simulink model "HybridControllerD3D3"  (Simulink 8.2)
settings: Solver=FixedStepDiscrete  StartTime=0.0  StopTime=inf  RelTol=1e-3
PreLoadFcn:
  | initializeSimulation
  | initializeSCRAMNetGT
values from neighbouring files (symbols this model uses):
  node = scgtnodestruct(node)    [initializeSCRAMNetGT.m]
undefined symbols (not defined in the file or in its folder): nAcc, nAct, nAdcU, nDucU, nTbl
undefined symbols (not defined in the file): controlPeriod, HybridCtrlParameters
libraries: xpclib x13, cwcec_scgtLib x7, simulink x4
CloseFcn:
  | rtwprivate ssgencode ModelCloseRequest scrnet_receiver
settings Model: Creator=aschellenberg  LastModifiedBy=RTHS Analyst  ExtModeArmWhenConnect=off  BufferReuse=off
settings DataIOCC: LimitDataPoints=off  SignalLoggingSaveFormat=Dataset  SaveOutput=off  SignalLogging=off  SaveTime=off  SignalLoggingName=sigsOut
settings OptimizationCC: BlockReduction=off  OptimizeBlockIOStorage=off  BufferReuse=off  ExpressionFolding=off  FoldNonRolledExpr=off  LocalBlockOutputs=off  UseTempVars=on  InitFltsAndDblsToZero=on  EfficientFloat2IntCast=on  SimCompilerOptimization=On
settings DebuggingCC: SaveWithParameterizedLinksMsg=none  CheckSSInitialOutputMsg=off  SolverPrmCheckMsg=none  FcnCallInpInsideContextMsg=EnableAllAsError
settings HardwareCC: ProdIntDivRoundTo=Zero  ProdEndianess=LittleEndian  ProdHWDeviceType=Generic->32-bit x86 compatible  TargetHWDeviceType=32-bit Generic
settings SFSimCC: SimCustomHeaderCode="#include \"PredictorCorrector.h\""  SimUserSources=PredictorCorrector.c  SimUserIncludeDirs="\"C:\\Program Files\\OpenFresco\\SourceCode\\SRC\\experimentalControl\\Simulink\\HybridSimToolbox\""
settings RTWCC: SystemTargetFile=xpctarget.tlc  TemplateMakefile=xpc_default_tmf  Description=xPC Target  ProcessScript=xpctarget_make_rtw_hook  CustomHeaderCode="#include \"PredictorCorrector.h\""  CustomInclude="\"C:\\Program Files\\OpenFresco\\SourceCode\\SRC\\experimentalControl\\Simulink\\HybridSimToolbox\""  CustomSource=PredictorCorrector.c  IncludeERTFirstTime=on  RTWCompilerOptimization=On
settings xpcTargetCC: TargetFcnLib=ansi_tfl_tmw.mat  CodeReplacementLibrary=XPC_BLAS  ParMdlRefBuildCompliant=on  ConcurrentExecutionCompliant=on  CombineSignalStateStructs=off  MATLABClassNameForMDSCustomization=xpcAperiodicCustomization  GRTInterface=on  GenerateAllocFcn=off  xPCTaskExecutionProfile=off  xPCRL32EventNumber=5000  RL32IRQSourceModifier=Auto (PCI only)  xPCIRQSourceBoard=SCRAMNet_GT200  xPCLoadParamSetFile=off  xPCConcurrentTasks=off  xPCEnableSFAnimation=off

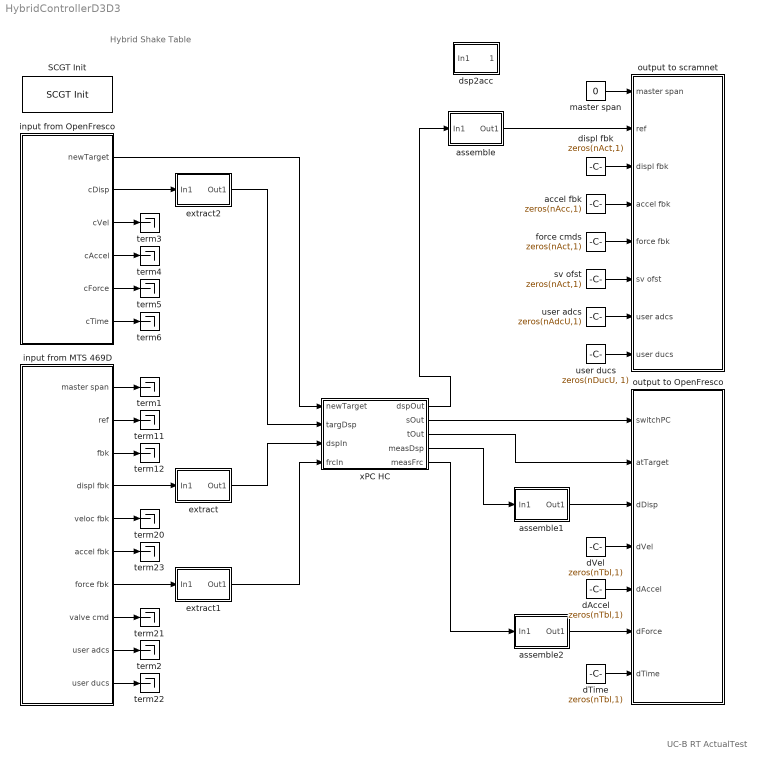
== system HybridControllerD3D3 ==
  note: Hybrid Shake Table
  note: UC-B RT ActualTest
  "SCGT Init " : cwcec_scgtLib/SCGT Init   node=node  pci=-1
  accel fbk : Constant  Value=zeros(nAcc,1)
  assemble : Subsystem  mask(to Actuators){id=[1], size=nTbl}
      mask prompts: id "Index Vector: id"; size "Vector Size: size"
      mask help: To select to which actuator(s) the signals are going to
      mask Display: disp('Assemble')
  assemble1 : Subsystem  mask(to Actuators){id=[1], size=nTbl}
      mask prompts: id "Index Vector: id"; size "Vector Size: size"
      mask help: To select to which actuator(s) the signals are going to
      mask Display: disp('Assemble')
  assemble2 : Subsystem  mask(to Actuators){id=[1], size=nTbl}
      mask prompts: id "Index Vector: id"; size "Vector Size: size"
      mask help: To select to which actuator(s) the signals are going to
      mask Display: disp('Assemble')
  dAccel : Constant  Value=zeros(nTbl,1)
  dTime : Constant  Value=zeros(nTbl,1)
  dVel : Constant  Value=zeros(nTbl,1)
  displ fbk : Constant  Value=zeros(nAct,1)
  dsp2acc : Subsystem
  extract : Subsystem  mask(from Actuators){id=[1], size=nTbl}
      mask prompts: id "Index Vector: id"; size "Vector Size: size"
      mask help: To select from which actuator(s) the signals are coming from
      mask Display: disp('Extract')
  extract1 : Subsystem  mask(from Actuators){id=[1], size=nTbl}
      mask prompts: id "Index Vector: id"; size "Vector Size: size"
      mask help: To select from which actuator(s) the signals are coming from
      mask Display: disp('Extract')
  extract2 : Subsystem  mask(from Actuators){id=[1], size=nTbl}
      mask prompts: id "Index Vector: id"; size "Vector Size: size"
      mask help: To select from which actuator(s) the signals are coming from
      mask Display: disp('Extract')
  force cmds : Constant  Value=zeros(nAct,1)
  input from MTS 469D : Subsystem
  input from OpenFresco : Subsystem
  master span : Constant  Value=0
  output to OpenFresco : Subsystem
  output to scramnet : Subsystem
  sv ofst : Constant  Value=zeros(nAct,1)
  term{1..6,11..12,20..23} (12 alike) : Terminator
  user adcs : Constant  Value=zeros(nAdcU,1)
  user ducs : Constant  Value=zeros(nDucU, 1)  OutDataTypeStr=uint32
  xPC HC : Subsystem  mask(Hybrid Controller: D3/D3){nAct=1, dtInt=HybridCtrlParameters.dtInt, dtSim=HybridCtrlParameters.dtSim, dtCon=HybridCtrlParameters.dtCon, N=HybridCtrlParameters.N, iDelay=HybridCtrlParameters.iDelay}
      mask prompts: nAct "Number of Actuators: nAct"; dtInt "Integration time step: dtInt"; dtSim "Simulation time step: dtSim"; dtCon "Controller time step: dtCon"; N "Maximum number of substeps: N"; iDelay "Number of delay steps: iDelay"
      mask help: Hybrid Controller using C0-continuous cubic Lagrange interpolation for prediction and correction
      mask Display: disp('xPC Target\nHybrid Controller\n(D3/D3)')
  wires:
  master span/1 -> output to scramnet/1(master span)
  force cmds/1 -> output to scramnet/5(force fbk)
  displ fbk/1 -> output to scramnet/3(displ fbk)
  user ducs/1 -> output to scramnet/8(user ducs)
  dVel/1 -> output to OpenFresco/4(dVel)
  dAccel/1 -> output to OpenFresco/5(dAccel)
  dTime/1 -> output to OpenFresco/7(dTime)
  input from OpenFresco/3(cVel) -> term3/1
  input from OpenFresco/5(cForce) -> term5/1
  input from OpenFresco/6(cTime) -> term6/1
  input from OpenFresco/1(newTarget) -> xPC HC/1(newTarget)
  extract2/1(Out1) -> xPC HC/2(targDsp)
  extract/1(Out1) -> xPC HC/3(dspIn)
  extract1/1(Out1) -> xPC HC/4(frcIn)
  xPC HC/1(dspOut) -> assemble/1(In1)
  xPC HC/5(measFrc) -> assemble2/1(In1)
  xPC HC/4(measDsp) -> assemble1/1(In1)
  xPC HC/3(tOut) -> output to OpenFresco/2(atTarget)
  xPC HC/2(sOut) -> output to OpenFresco/1(switchPC)
  assemble1/1(Out1) -> output to OpenFresco/3(dDisp)
  assemble2/1(Out1) -> output to OpenFresco/6(dForce)
  input from MTS 469D/1(master span) -> term1/1
  input from MTS 469D/2(ref) -> term11/1
  input from MTS 469D/3(fbk) -> term12/1
  input from MTS 469D/4(displ fbk) -> extract/1(In1)
  input from MTS 469D/5(veloc fbk) -> term20/1
  input from MTS 469D/6(accel fbk) -> term23/1
  input from MTS 469D/7(force fbk) -> extract1/1(In1)
  input from MTS 469D/8(valve cmd) -> term21/1
  input from MTS 469D/10(user ducs) -> term22/1
  input from MTS 469D/9(user adcs) -> term2/1
  accel fbk/1 -> output to scramnet/4(accel fbk)
  user adcs/1 -> output to scramnet/7(user adcs)
  input from OpenFresco/2(cDisp) -> extract2/1(In1)
  input from OpenFresco/4(cAccel) -> term4/1
  sv ofst/1 -> output to scramnet/6(sv ofst)
  assemble/1(Out1) -> output to scramnet/2(ref)

== system HybridControllerD3D3/assemble ==
  In1 : Inport
  Assignment : Assignment  OutputInitialize=Specify size for each dimension in table  IndexOptions=Index vector (port)  Indices=1  OutputSizes=size
  Constant : Constant  Value=id
  Out1 : Outport
  wires:
  Constant/1 -> Assignment/2
  Assignment/1 -> Out1/1
  In1/1 -> Assignment/1

== system HybridControllerD3D3/assemble1 ==
  In1 : Inport
  Assignment : Assignment  OutputInitialize=Specify size for each dimension in table  IndexOptions=Index vector (port)  Indices=1  OutputSizes=size
  Constant : Constant  Value=id
  Out1 : Outport
  wires:
  Constant/1 -> Assignment/2
  Assignment/1 -> Out1/1
  In1/1 -> Assignment/1

== system HybridControllerD3D3/assemble2 ==
  In1 : Inport
  Assignment : Assignment  OutputInitialize=Specify size for each dimension in table  IndexOptions=Index vector (port)  Indices=1  OutputSizes=size
  Constant : Constant  Value=id
  Out1 : Outport
  wires:
  Constant/1 -> Assignment/2
  Assignment/1 -> Out1/1
  In1/1 -> Assignment/1

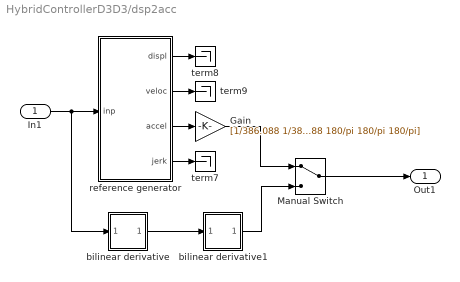
== system HybridControllerD3D3/dsp2acc ==
  In1 : Inport
  Gain : Gain  Gain=[1/386.088 1/386.088 1/386.088 180/pi 180/pi 180/pi]
  Manual Switch : ManualSwitch
  bilinear derivative : Subsystem  mask(Discrete Bilinear Differentiator){decay=1, initialCondition=0, samplePeriod=controlPeriod}
      mask prompts: decay "Decay time constant (0: backward Euler, 1: binlinear)"; initialCondition "Initial condition"; samplePeriod "Sample period"
      mask Display:
      | text(0.1,.75,'2');
      | text(0.1,.65,'_');
      | text(0.1,.25,'T');
      | text(.3,.80,'{1-z}^{-1}', 'hor','left','texmode','on');
      | text(.3,.65,'___');
      | text(.3,.30,'{1+z}^{-1}', 'hor','left','texmode','on');
  bilinear derivative1 : Subsystem  mask(Discrete Bilinear Differentiator){decay=1, initialCondition=0, samplePeriod=controlPeriod}
      mask prompts: decay "Decay time constant (0: backward Euler, 1: binlinear)"; initialCondition "Initial condition"; samplePeriod "Sample period"
      mask Display:
      | text(0.1,.75,'2');
      | text(0.1,.65,'_');
      | text(0.1,.25,'T');
      | text(.3,.80,'{1-z}^{-1}', 'hor','left','texmode','on');
      | text(.3,.65,'___');
      | text(.3,.30,'{1+z}^{-1}', 'hor','left','texmode','on');
  reference generator : Subsystem  mask(Reference Generator){mode=1, freqHP=0.0625, freqLP=128, displCanon=1, velocCanon=1, accelCanon=1, jerkCanon=1, samplePeriod=controlPeriod}
      mask prompts: mode "Mode (1: displ, 2: veloc, 3: accel)"; freqHP "Cut-in frequency (Hz)"; freqLP "Cutoff frequency (Hz)"; displCanon "Canonical displacement units"; velocCanon "Canonical velocity units"; accelCanon "Canonical acceleration units"; jerkCanon "Canonical jerk units"; samplePeriod "Sample period (sec)"
      mask init:
      | omegaHP	= 2 * pi * freqHP;
      | omegaLP	= 2 * pi * freqLP;
      | if mode == 1
      | 	damp = 0.707106781186547;
      | 	b  = omegaLP * omegaLP;
      | 	a0 = 0;
      | 	a1 = omegaLP * omegaLP;
      | 	a2 = 2 * damp * omegaLP;
      | 	canon = displCanon;
      | elseif mode == 2
      | 	damp = 0.707106781186547;
      | 	b  = omegaLP;
      | 	a0 = omegaHP * omegaHP * omegaLP;
      | 	a1 = (2 * damp * omegaLP + omegaHP) * omegaHP;
      | 	a2 = 2 * damp * omegaHP + omegaLP;
      | 	canon = velocCanon;
      | elseif mode == 3
      | 	damp = 0.5;
      | 	b  = 1;
      | 	a0 = omegaHP * omegaHP * omegaHP;
      | 	a1 = (2 * damp + 1) * omegaHP * omegaHP;
      | 	a2 = (2 * damp + 1) * omegaHP;
      | 	canon = accelCanon;
      | end
  term7 : Terminator
  term8 : Terminator
  term9 : Terminator
  Out1 : Outport
  wires:
  In1/1 -> reference generator/1(inp), bilinear derivative/1(inp)
  reference generator/2(veloc) -> term9/1
  reference generator/4(jerk) -> term7/1
  reference generator/1(displ) -> term8/1
  reference generator/3(accel) -> Gain/1
  bilinear derivative/1(out) -> bilinear derivative1/1(inp)
  Gain/1 -> Manual Switch/1
  bilinear derivative1/1(out) -> Manual Switch/2
  Manual Switch/1 -> Out1/1

== system HybridControllerD3D3/extract ==
  In1 : Inport
  Selector : Selector  InputPortWidth=size  IndexOptions=Index vector (dialog)  Indices=id  OutputSizes=1
  Out1 : Outport
  wires:
  Selector/1 -> Out1/1
  In1/1 -> Selector/1

== system HybridControllerD3D3/extract1 ==
  In1 : Inport
  Selector : Selector  InputPortWidth=size  IndexOptions=Index vector (dialog)  Indices=id  OutputSizes=1
  Out1 : Outport
  wires:
  Selector/1 -> Out1/1
  In1/1 -> Selector/1

== system HybridControllerD3D3/extract2 ==
  In1 : Inport
  Selector : Selector  InputPortWidth=size  IndexOptions=Index vector (dialog)  Indices=id  OutputSizes=1
  Out1 : Outport
  wires:
  Selector/1 -> Out1/1
  In1/1 -> Selector/1

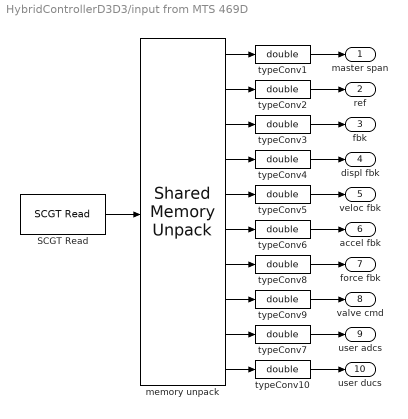
== system HybridControllerD3D3/input from MTS 469D ==
  "SCGT Read " : cwcec_scgtLib/SCGT Read   partition=node.Partitions(9:18)  ts=controlPeriod  pci=-1
  memory unpack : xpclib/Shared Memory/Shared Memory Unpack   partition=node.Partitions(9:18)
  typeConv{1..10} (10 alike) : DataTypeConversion  OutDataTypeStr=double  SaturateOnIntegerOverflow=on  RndMeth=Zero
  master span : Outport
  ref : Outport  Port=2
  fbk : Outport  Port=3
  displ fbk : Outport  Port=4
  veloc fbk : Outport  Port=5
  accel fbk : Outport  Port=6
  force fbk : Outport  Port=7
  valve cmd : Outport  Port=8
  user adcs : Outport  Port=9
  user ducs : Outport  Port=10
  wires:
  memory unpack/10 -> typeConv10/1
  memory unpack/9 -> typeConv7/1
  memory unpack/8 -> typeConv9/1
  memory unpack/7 -> typeConv8/1
  memory unpack/6 -> typeConv6/1
  memory unpack/5 -> typeConv5/1
  memory unpack/4 -> typeConv4/1
  memory unpack/3 -> typeConv3/1
  memory unpack/2 -> typeConv2/1
  memory unpack/1 -> typeConv1/1
  typeConv2/1 -> ref/1
  typeConv1/1 -> master span/1
  "SCGT Read "/1 -> memory unpack/1
  typeConv3/1 -> fbk/1
  typeConv4/1 -> displ fbk/1
  typeConv5/1 -> veloc fbk/1
  typeConv6/1 -> accel fbk/1
  typeConv8/1 -> force fbk/1
  typeConv9/1 -> valve cmd/1
  typeConv7/1 -> user adcs/1
  typeConv10/1 -> user ducs/1

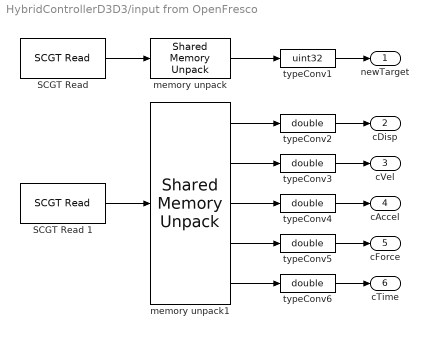
== system HybridControllerD3D3/input from OpenFresco ==
  "SCGT Read " : cwcec_scgtLib/SCGT Read   partition=node.Partitions(19)  ts=controlPeriod  pci=-1
  SCGT Read 1 : cwcec_scgtLib/SCGT Read   partition=node.Partitions(22:26)  ts=controlPeriod  pci=-1
  memory unpack : xpclib/Shared Memory/Shared Memory Unpack   partition=node.Partitions(19)
  memory unpack1 : xpclib/Shared Memory/Shared Memory Unpack   partition=node.Partitions(22:26)
  typeConv1 : DataTypeConversion  OutDataTypeStr=uint32  SaturateOnIntegerOverflow=on  RndMeth=Zero
  typeConv{2..6} (5 alike) : DataTypeConversion  OutDataTypeStr=double  SaturateOnIntegerOverflow=on  RndMeth=Zero
  newTarget : Outport
  cDisp : Outport  Port=2
  cVel : Outport  Port=3
  cAccel : Outport  Port=4
  cForce : Outport  Port=5
  cTime : Outport  Port=6
  wires:
  typeConv1/1 -> newTarget/1
  memory unpack/1 -> typeConv1/1
  typeConv2/1 -> cDisp/1
  typeConv3/1 -> cVel/1
  memory unpack1/2 -> typeConv3/1
  typeConv4/1 -> cAccel/1
  memory unpack1/3 -> typeConv4/1
  typeConv5/1 -> cForce/1
  typeConv6/1 -> cTime/1
  memory unpack1/5 -> typeConv6/1
  memory unpack1/4 -> typeConv5/1
  "SCGT Read "/1 -> memory unpack/1
  SCGT Read 1/1 -> memory unpack1/1
  memory unpack1/1 -> typeConv2/1

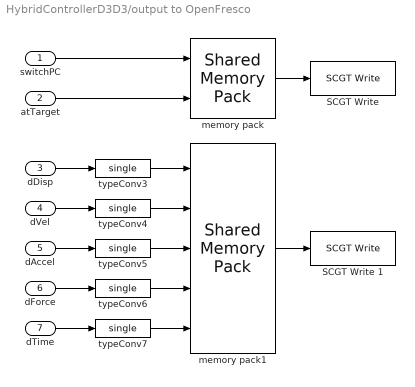
== system HybridControllerD3D3/output to OpenFresco ==
  switchPC : Inport
  atTarget : Inport  Port=2
  dDisp : Inport  Port=3
  dVel : Inport  Port=4
  dAccel : Inport  Port=5
  dForce : Inport  Port=6
  dTime : Inport  Port=7
  "SCGT Write " : cwcec_scgtLib/SCGT Write   partition=node.Partitions(20:21)  ts=controlPeriod  pci=-1
  SCGT Write 1 : cwcec_scgtLib/SCGT Write   partition=node.Partitions(27:31)  ts=controlPeriod  pci=-1
  memory pack : xpclib/Shared Memory/Shared Memory Pack   partition=node.Partitions(20:21)
  memory pack1 : xpclib/Shared Memory/Shared Memory Pack   partition=node.Partitions(27:31)
  typeConv{3..7} (5 alike) : DataTypeConversion  OutDataTypeStr=single  SaturateOnIntegerOverflow=on  RndMeth=Zero
  wires:
  dAccel/1 -> typeConv5/1
  switchPC/1 -> memory pack/1
  dVel/1 -> typeConv4/1
  dDisp/1 -> typeConv3/1
  typeConv4/1 -> memory pack1/2
  typeConv5/1 -> memory pack1/3
  dForce/1 -> typeConv6/1
  typeConv6/1 -> memory pack1/4
  dTime/1 -> typeConv7/1
  typeConv7/1 -> memory pack1/5
  atTarget/1 -> memory pack/2
  memory pack/1 -> "SCGT Write "/1
  memory pack1/1 -> SCGT Write 1/1
  typeConv3/1 -> memory pack1/1

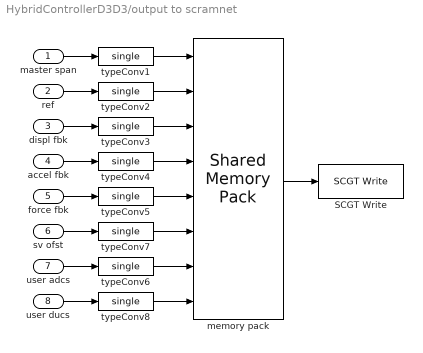
== system HybridControllerD3D3/output to scramnet ==
  master span : Inport
  ref : Inport  Port=2
  displ fbk : Inport  Port=3
  accel fbk : Inport  Port=4
  force fbk : Inport  Port=5
  sv ofst : Inport  Port=6
  user adcs : Inport  Port=7
  user ducs : Inport  Port=8
  "SCGT Write " : cwcec_scgtLib/SCGT Write   partition=node.Partitions(1:8)  ts=controlPeriod  pci=-1
  memory pack : xpclib/Shared Memory/Shared Memory Pack   partition=node.Partitions(1:8)
  typeConv{1..8} (8 alike) : DataTypeConversion  OutDataTypeStr=single  SaturateOnIntegerOverflow=on  RndMeth=Zero
  wires:
  typeConv8/1 -> memory pack/8
  user ducs/1 -> typeConv8/1
  user adcs/1 -> typeConv6/1
  sv ofst/1 -> typeConv7/1
  master span/1 -> typeConv1/1
  ref/1 -> typeConv2/1
  displ fbk/1 -> typeConv3/1
  accel fbk/1 -> typeConv4/1
  memory pack/1 -> "SCGT Write "/1
  typeConv1/1 -> memory pack/1
  typeConv2/1 -> memory pack/2
  typeConv3/1 -> memory pack/3
  typeConv4/1 -> memory pack/4
  force fbk/1 -> typeConv5/1
  typeConv5/1 -> memory pack/5
  typeConv7/1 -> memory pack/6
  typeConv6/1 -> memory pack/7

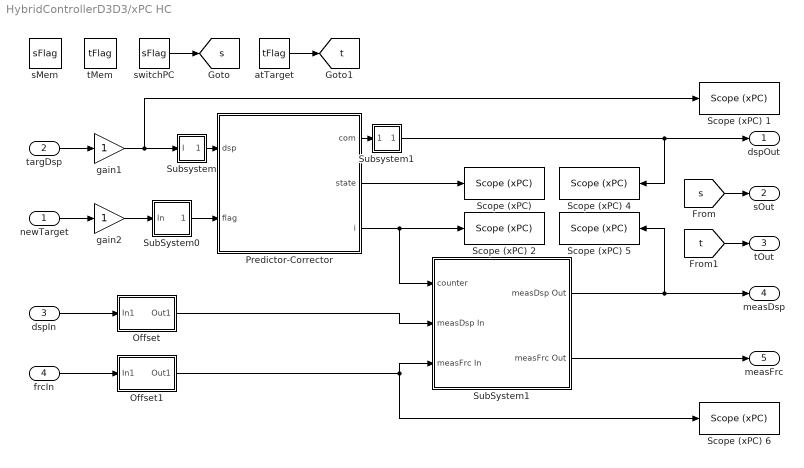
== system HybridControllerD3D3/xPC HC ==
  newTarget : Inport
  targDsp : Inport  Port=2
  dspIn : Inport  Port=3
  frcIn : Inport  Port=4
  Offset : Subsystem  mask(Signal Offset){nS=nAct, nOffset=1/dtCon, dt=dtCon}
      mask prompts: nS "Number of Signals: nS"; nOffset "Number of samples to initialize offset: nOffset"; dt "Sample time: dt"
      mask help: Offset signal by average of signal over initial number of samples
      mask Display: fprintf('Signal\nOffset')
  Offset1 : Subsystem  mask(Signal Offset){nS=nAct, nOffset=1/dtCon, dt=dtCon}
      mask prompts: nS "Number of Signals: nS"; nOffset "Number of samples to initialize offset: nOffset"; dt "Sample time: dt"
      mask help: Offset signal by average of signal over initial number of samples
      mask Display: fprintf('Signal\nOffset')
  Predictor-Corrector : Stateflow chart  TreatAsAtomicUnit=on
  "Scope (xPC) " : xpclib/Misc./Scope (xPC)   scopeno=4  scopetype=File  autostart=on  viewmode=Graphical redraw  formatstr='%15.6f'  grid=on  ylimits=[0,3]  nosamples=4096  noprepostsamples=0  interleave=1  triggermode=FreeRun  triggersignal=1  trigsignalfromport=off  triggerlevel=0.0  triggerslope=Either  triggerscope=1  triggersample=0  filename=D:\state.dat  mode=Lazy  writesize=512  autorestart=on  dynamicfilemode=off  maxwritefilesize=512*1024^2
  Scope (xPC) 1 : xpclib/Misc./Scope (xPC)   scopeno=1  scopetype=File  autostart=on  viewmode=Numerical  formatstr='%15.6f'  grid=on  ylimits=[-4,4]  nosamples=4096  noprepostsamples=0  interleave=1  triggermode=FreeRun  triggersignal=1  trigsignalfromport=off  triggerlevel=0.0  triggerslope=Either  triggerscope=1  triggersample=0  filename=D:\targDsp.dat  mode=Lazy  writesize=512  autorestart=on  dynamicfilemode=off  maxwritefilesize=512*1024^2
  Scope (xPC) 2 : xpclib/Misc./Scope (xPC)   scopeno=5  scopetype=File  autostart=on  viewmode=Numerical  formatstr='%15.6f'  grid=on  ylimits=[0,3]  nosamples=4096  noprepostsamples=0  interleave=1  triggermode=FreeRun  triggersignal=1  trigsignalfromport=off  triggerlevel=0.0  triggerslope=Either  triggerscope=1  triggersample=0  filename=D:\count.dat  mode=Lazy  writesize=512  autorestart=on  dynamicfilemode=off  maxwritefilesize=512*1024^2
  Scope (xPC) 4 : xpclib/Misc./Scope (xPC)   scopeno=2  scopetype=File  autostart=on  viewmode=Numerical  formatstr='%15.6f'  grid=on  ylimits=[-4,4]  nosamples=4096  noprepostsamples=0  interleave=1  triggermode=FreeRun  triggersignal=1  trigsignalfromport=off  triggerlevel=0.0  triggerslope=Either  triggerscope=1  triggersample=0  filename=D:\commDsp.dat  mode=Lazy  writesize=512  autorestart=on  dynamicfilemode=off  maxwritefilesize=512*1024^2
  Scope (xPC) 5 : xpclib/Misc./Scope (xPC)   scopeno=3  scopetype=File  autostart=on  viewmode=Numerical  formatstr='%15.6f'  grid=on  ylimits=[-4,4]  nosamples=4096  noprepostsamples=0  interleave=1  triggermode=FreeRun  triggersignal=1  trigsignalfromport=off  triggerlevel=0.0  triggerslope=Either  triggerscope=1  triggersample=0  filename=D:\measDsp.dat  mode=Lazy  writesize=512  autorestart=on  dynamicfilemode=off  maxwritefilesize=512*1024^2
  Scope (xPC) 6 : xpclib/Misc./Scope (xPC)   scopeno=6  scopetype=File  autostart=on  viewmode=Numerical  formatstr='%15.6f'  grid=on  ylimits=[0,3]  nosamples=4096  noprepostsamples=0  interleave=1  triggermode=FreeRun  triggersignal=1  trigsignalfromport=off  triggerlevel=0.0  triggerslope=Either  triggerscope=1  triggersample=0  filename=D:\measFrc.dat  mode=Lazy  writesize=512  autorestart=on  dynamicfilemode=off  maxwritefilesize=512*1024^2
  SubSystem0 : Subsystem
  SubSystem1 : Subsystem
  Subsystem : Subsystem
      mask Display: disp('I/O')
  Subsystem1 : Subsystem
      mask Display: disp('I/O')
  atTarget : DataStoreRead  DataStoreName=tFlag  SampleTime=dtCon
  gain1 : Gain  OutDataTypeStr=Inherit: Same as input
  gain2 : Gain  OutDataTypeStr=Inherit: Same as input  ParamDataTypeStr=Inherit: Same as input
  sMem : DataStoreMemory  DataStoreName=sFlag  OutDataTypeStr=uint32
  switchPC : DataStoreRead  DataStoreName=sFlag  SampleTime=dtCon
  tMem : DataStoreMemory  DataStoreName=tFlag  OutDataTypeStr=uint32
  dspOut : Outport
  sOut : Outport  Port=2
  tOut : Outport  Port=3
  measDsp : Outport  Port=4
  measFrc : Outport  Port=5
  tag scope: s=global, t=global
  wires:
  frcIn/1 -> Offset1/1(In1)
  dspIn/1 -> Offset/1(In1)
  SubSystem1/2(measFrc Out) -> measFrc/1
  SubSystem1/1(measDsp Out) -> Scope (xPC) 5/1, measDsp/1
  Predictor-Corrector/3(i) -> SubSystem1/1(counter), Scope (xPC) 2/1
  Predictor-Corrector/2(state) -> "Scope (xPC) "/1
  Predictor-Corrector/1(com) -> Subsystem1/1(In)
  Offset/1(Out1) -> SubSystem1/2(measDsp In)
  SubSystem0/1(Out) -> Predictor-Corrector/2(flag)
  newTarget/1 -> gain2/1
  switchPC/1 -> [s]
  atTarget/1 -> [t]
  targDsp/1 -> gain1/1
  Offset1/1(Out1) -> Scope (xPC) 6/1, SubSystem1/3(measFrc In)
  [s] -> sOut/1
  [t] -> tOut/1
  gain1/1 -> Scope (xPC) 1/1, Subsystem/1(I)
  gain2/1 -> SubSystem0/1(In)
  Subsystem1/1(Out) -> Scope (xPC) 4/1, dspOut/1
  Subsystem/1(O) -> Predictor-Corrector/1(dsp)

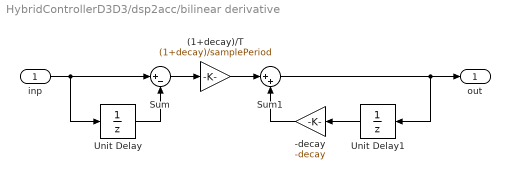
== system HybridControllerD3D3/dsp2acc/bilinear derivative ==
  inp : Inport
  (1+decay)/T : Gain  Gain=(1+decay)/samplePeriod
  -decay : Gain  Gain=-decay
  Sum : Sum  Inputs=|+-  SaturateOnIntegerOverflow=on  InputSameDT=on  OutDataTypeStr=Inherit: Same as first input
  Sum1 : Sum  Inputs=|++  SaturateOnIntegerOverflow=on  InputSameDT=on  OutDataTypeStr=Inherit: Same as first input
  Unit Delay : UnitDelay  InitialCondition=initialCondition  SampleTime=-1
  Unit Delay1 : UnitDelay  SampleTime=-1
  out : Outport
  wires:
  Sum/1 -> (1+decay)/T/1
  Unit Delay1/1 -> -decay/1
  inp/1 -> Sum/1, Unit Delay/1
  Unit Delay/1 -> Sum/2
  -decay/1 -> Sum1/2
  Sum1/1 -> out/1, Unit Delay1/1
  (1+decay)/T/1 -> Sum1/1

== system HybridControllerD3D3/dsp2acc/bilinear derivative1 ==
  inp : Inport
  (1+decay)/T : Gain  Gain=(1+decay)/samplePeriod
  -decay : Gain  Gain=-decay
  Sum : Sum  Inputs=|+-  SaturateOnIntegerOverflow=on  InputSameDT=on  OutDataTypeStr=Inherit: Same as first input
  Sum1 : Sum  Inputs=|++  SaturateOnIntegerOverflow=on  InputSameDT=on  OutDataTypeStr=Inherit: Same as first input
  Unit Delay : UnitDelay  InitialCondition=initialCondition  SampleTime=-1
  Unit Delay1 : UnitDelay  SampleTime=-1
  out : Outport
  wires:
  Sum/1 -> (1+decay)/T/1
  Unit Delay1/1 -> -decay/1
  inp/1 -> Sum/1, Unit Delay/1
  Unit Delay/1 -> Sum/2
  -decay/1 -> Sum1/2
  Sum1/1 -> out/1, Unit Delay1/1
  (1+decay)/T/1 -> Sum1/1

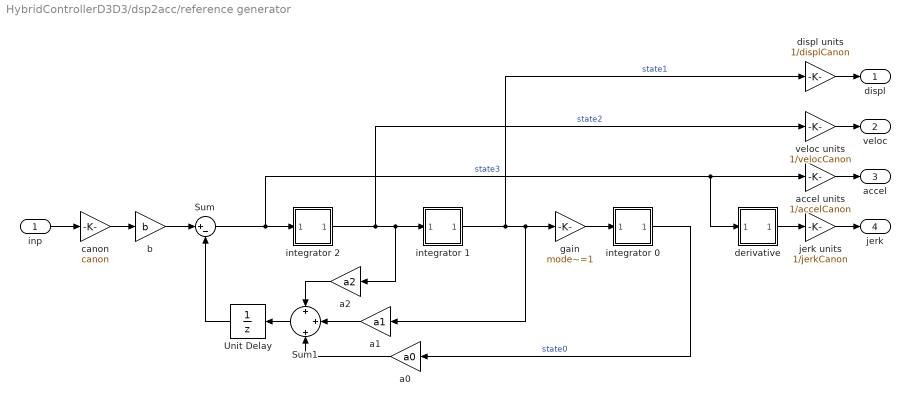
== system HybridControllerD3D3/dsp2acc/reference generator ==
  inp : Inport
  Sum : Sum  Inputs=|+-
  Sum1 : Sum  Inputs=+|+|+
  Unit Delay : UnitDelay  SampleTime=-1
  a0 : Gain  Gain=a0
  a1 : Gain  Gain=a1
  a2 : Gain  Gain=a2
  accel units : Gain  Gain=1/accelCanon
  b : Gain  Gain=b
  canon : Gain  Gain=canon
  derivative : Subsystem  mask(Discrete Euler Derivative){initialCondition=0, samplePeriod=samplePeriod}
      mask prompts: initialCondition "Initial condition"; samplePeriod "Sample period (sec)"
      mask Display: dpoly([1 -1], '[T]', 'z-')
  displ units : Gain  Gain=1/displCanon
  gain : Gain  Gain=mode~=1
  integrator 0 : Subsystem  mask(Discrete Bilinear Integrator){initialCondition=0, samplePeriod=samplePeriod}
      mask prompts: initialCondition "Initial condition"; samplePeriod "Sample period (sec)"
      mask Display:
      | text(0.1,.75,'T');
      | text(0.1,.65,'_');
      | text(0.1,.25,'2');
      | text(.3,.80,'{1+z}^{-1}', 'hor','left','texmode','on');
      | text(.3,.65,'___');
      | text(.3,.30,'{1-z}^{-1}', 'hor','left','texmode','on');
  integrator 1 : Subsystem  mask(Discrete Bilinear Integrator){initialCondition=0, samplePeriod=samplePeriod}
      mask prompts: initialCondition "Initial condition"; samplePeriod "Sample period (sec)"
      mask Display:
      | text(0.1,.75,'T');
      | text(0.1,.65,'_');
      | text(0.1,.25,'2');
      | text(.3,.80,'{1+z}^{-1}', 'hor','left','texmode','on');
      | text(.3,.65,'___');
      | text(.3,.30,'{1-z}^{-1}', 'hor','left','texmode','on');
  integrator 2 : Subsystem  mask(Discrete Bilinear Integrator){initialCondition=0, samplePeriod=samplePeriod}
      mask prompts: initialCondition "Initial condition"; samplePeriod "Sample period (sec)"
      mask Display:
      | text(0.1,.75,'T');
      | text(0.1,.65,'_');
      | text(0.1,.25,'2');
      | text(.3,.80,'{1+z}^{-1}', 'hor','left','texmode','on');
      | text(.3,.65,'___');
      | text(.3,.30,'{1-z}^{-1}', 'hor','left','texmode','on');
  jerk units : Gain  Gain=1/jerkCanon
  veloc units : Gain  Gain=1/velocCanon
  displ : Outport
  veloc : Outport  Port=2
  accel : Outport  Port=3
  jerk : Outport  Port=4
  wires:
  gain/1 -> integrator 0/1(inp)
  derivative/1(out) -> jerk units/1
  Unit Delay/1 -> Sum/2
  jerk units/1 -> jerk/1
  canon/1 -> b/1
  displ units/1 -> displ/1
  veloc units/1 -> veloc/1
  accel units/1 -> accel/1
  inp/1 -> canon/1
  integrator 0/1(out) -> a0/1  "state0"
  a0/1 -> Sum1/3
  a1/1 -> Sum1/2
  a2/1 -> Sum1/1
  Sum1/1 -> Unit Delay/1
  b/1 -> Sum/1
  Sum/1 -> integrator 2/1(inp), derivative/1(inp), accel units/1  "state3"
  integrator 1/1(out) -> displ units/1, gain/1, a1/1  "state1"
  integrator 2/1(out) -> veloc units/1, integrator 1/1(inp), a2/1  "state2"

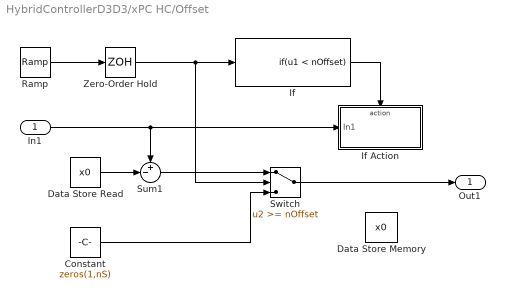
== system HybridControllerD3D3/xPC HC/Offset ==
  In1 : Inport
  Constant : Constant  Value=zeros(1,nS)
  Data Store Memory : DataStoreMemory  DataStoreName=x0  InitialValue=zeros(1,nS)  OutDataTypeStr=double
  Data Store Read : DataStoreRead  DataStoreName=x0  SampleTime=dt
  If : If  IfExpression=u1 < nOffset  ShowElse=off
  If Action : Subsystem  TreatAsAtomicUnit=on
  Ramp : simulink/Sources/Ramp  slope=1/dt  start=0  X0=0
  Sum1 : Sum  Inputs=+-|  SaturateOnIntegerOverflow=on  InputSameDT=on  OutDataTypeStr=Inherit: Same as first input
  Switch : Switch  Threshold=nOffset  SaturateOnIntegerOverflow=on  InputSameDT=on
  Zero-Order Hold : ZeroOrderHold  SampleTime=dt
  Out1 : Outport
  wires:
  Switch/1 -> Out1/1
  Sum1/1 -> Switch/1
  Data Store Read/1 -> Sum1/2
  In1/1 -> If Action/1(In1), Sum1/1
  Constant/1 -> Switch/3
  Zero-Order Hold/1 -> Switch/2, If/1
  If/1 -> If Action/Action
  Ramp/1 -> Zero-Order Hold/1

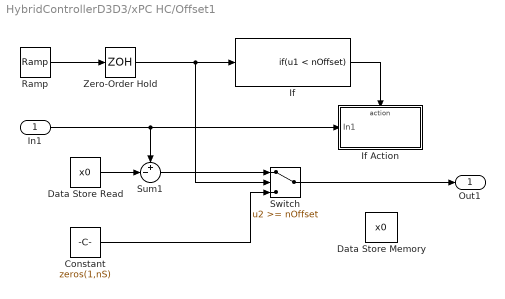
== system HybridControllerD3D3/xPC HC/Offset1 ==
  In1 : Inport
  Constant : Constant  Value=zeros(1,nS)
  Data Store Memory : DataStoreMemory  DataStoreName=x0  InitialValue=zeros(1,nS)  OutDataTypeStr=double
  Data Store Read : DataStoreRead  DataStoreName=x0  SampleTime=dt
  If : If  IfExpression=u1 < nOffset  ShowElse=off
  If Action : Subsystem  TreatAsAtomicUnit=on
  Ramp : simulink/Sources/Ramp  slope=1/dt  start=0  X0=0
  Sum1 : Sum  Inputs=+-|  SaturateOnIntegerOverflow=on  InputSameDT=on  OutDataTypeStr=Inherit: Same as first input
  Switch : Switch  Threshold=nOffset  SaturateOnIntegerOverflow=on  InputSameDT=on
  Zero-Order Hold : ZeroOrderHold  SampleTime=dt
  Out1 : Outport
  wires:
  Switch/1 -> Out1/1
  Sum1/1 -> Switch/1
  Data Store Read/1 -> Sum1/2
  In1/1 -> If Action/1(In1), Sum1/1
  Constant/1 -> Switch/3
  Zero-Order Hold/1 -> Switch/2, If/1
  If/1 -> If Action/Action
  Ramp/1 -> Zero-Order Hold/1

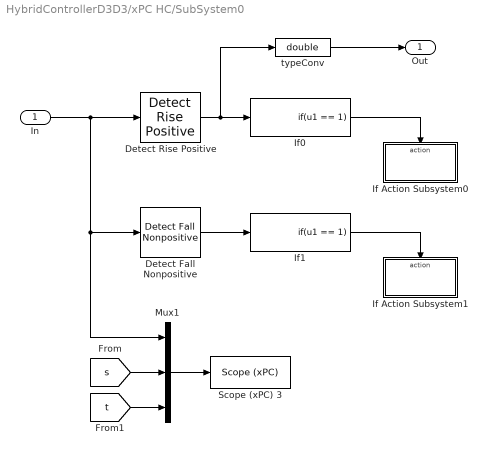
== system HybridControllerD3D3/xPC HC/SubSystem0 ==
  In : Inport
  Detect Fall Nonpositive : simulink/Logic and Bit Operations/Detect Fall Nonpositive  vinit=0  InputProcessing=Inherited  OutDataTypeStr=uint8
  Detect Rise Positive : simulink/Logic and Bit Operations/Detect Rise Positive  vinit=0  InputProcessing=Inherited  OutDataTypeStr=uint8
  If Action Subsystem0 : Subsystem  TreatAsAtomicUnit=on
  If Action Subsystem1 : Subsystem  TreatAsAtomicUnit=on
  If0 : If  IfExpression=u1 == 1  ShowElse=off
  If1 : If  IfExpression=u1 == 1  ShowElse=off
  Mux1 : Mux  Inputs=3
  Scope (xPC) 3 : xpclib/Misc./Scope (xPC)   scopeno=7  scopetype=File  autostart=on  viewmode=Numerical  formatstr='%15.6f'  grid=on  ylimits=[0,3]  nosamples=4096  noprepostsamples=0  interleave=1  triggermode=FreeRun  triggersignal=1  trigsignalfromport=off  triggerlevel=0.0  triggerslope=Either  triggerscope=1  triggersample=0  filename=D:\flag.dat  mode=Lazy  writesize=512  autorestart=on  dynamicfilemode=off  maxwritefilesize=512*1024^2
  typeConv : DataTypeConversion  OutDataTypeStr=double  SaturateOnIntegerOverflow=on  RndMeth=Zero
  Out : Outport
  wires:
  In/1 -> Detect Rise Positive/1, Detect Fall Nonpositive/1, Mux1/1
  Detect Rise Positive/1 -> If0/1, typeConv/1
  Detect Fall Nonpositive/1 -> If1/1
  If1/1 -> If Action Subsystem1/Action
  If0/1 -> If Action Subsystem0/Action
  typeConv/1 -> Out/1
  Mux1/1 -> Scope (xPC) 3/1
  [s] -> Mux1/2
  [t] -> Mux1/3

== system HybridControllerD3D3/xPC HC/SubSystem1 ==
  counter : Inport
  measDsp In : Inport  Port=2
  measFrc In : Inport  Port=3
  SubSystem : Subsystem  TreatAsAtomicUnit=on
  Subsystem : Subsystem
  measDsp Out : Outport
  measFrc Out : Outport  Port=2
  wires:
  SubSystem/2(measFrc Out) -> measFrc Out/1
  measFrc In/1 -> SubSystem/2(measFrc In)
  SubSystem/1(measDsp Out) -> measDsp Out/1
  measDsp In/1 -> SubSystem/1(measDsp In)
  counter/1 -> Subsystem/1(i)
  Subsystem/1(trig) -> SubSystem/Trigger

== system HybridControllerD3D3/xPC HC/Subsystem ==
  I : Inport  PortDimensions=nAct
  Dummy Aug : Mux  Inputs=[nAct 1]
  Dummy Zero : Constant  Value=0  OutDataTypeStr=double  SampleTime=dtCon
  O : Outport  PortDimensions=nAct+1
  wires:
  Dummy Zero/1 -> Dummy Aug/2
  I/1 -> Dummy Aug/1
  Dummy Aug/1 -> O/1

== system HybridControllerD3D3/xPC HC/Subsystem1 ==
  In : Inport  PortDimensions=nAct+1
  Dummy Trn : Demux  Outputs=[nAct 1]
  Terminator3 : Terminator
  Out : Outport  PortDimensions=nAct
  wires:
  Dummy Trn/2 -> Terminator3/1
  Dummy Trn/1 -> Out/1
  In/1 -> Dummy Trn/1

== system HybridControllerD3D3/dsp2acc/reference generator/derivative ==
  inp : Inport
  1/T : Gain  Gain=1/samplePeriod
  Sum : Sum  Inputs=|+-  SaturateOnIntegerOverflow=on  InputSameDT=on  OutDataTypeStr=Inherit: Same as first input
  Unit Delay : UnitDelay  InitialCondition=initialCondition  SampleTime=-1
  out : Outport
  wires:
  1/T/1 -> out/1
  Unit Delay/1 -> Sum/2
  inp/1 -> Sum/1, Unit Delay/1
  Sum/1 -> 1/T/1

== system HybridControllerD3D3/dsp2acc/reference generator/integrator 0 ==
  inp : Inport
  Sum : Sum  Inputs=|++  SaturateOnIntegerOverflow=on  InputSameDT=on  OutDataTypeStr=Inherit: Same as first input
  Sum1 : Sum  Inputs=|++  SaturateOnIntegerOverflow=on  InputSameDT=on  OutDataTypeStr=Inherit: Same as first input
  T/2 : Gain  Gain=samplePeriod/2
  Unit Delay : UnitDelay  SampleTime=-1
  Unit Delay1 : UnitDelay  InitialCondition=initialCondition  SampleTime=-1
  out : Outport
  wires:
  T/2/1 -> Sum1/1
  Sum1/1 -> out/1, Unit Delay1/1
  Unit Delay1/1 -> Sum1/2
  Unit Delay/1 -> Sum/2
  inp/1 -> Sum/1, Unit Delay/1
  Sum/1 -> T/2/1

== system HybridControllerD3D3/dsp2acc/reference generator/integrator 1 ==
  inp : Inport
  Sum : Sum  Inputs=|++  SaturateOnIntegerOverflow=on  InputSameDT=on  OutDataTypeStr=Inherit: Same as first input
  Sum1 : Sum  Inputs=|++  SaturateOnIntegerOverflow=on  InputSameDT=on  OutDataTypeStr=Inherit: Same as first input
  T/2 : Gain  Gain=samplePeriod/2
  Unit Delay : UnitDelay  SampleTime=-1
  Unit Delay1 : UnitDelay  InitialCondition=initialCondition  SampleTime=-1
  out : Outport
  wires:
  T/2/1 -> Sum1/1
  Sum1/1 -> out/1, Unit Delay1/1
  Unit Delay1/1 -> Sum1/2
  Unit Delay/1 -> Sum/2
  inp/1 -> Sum/1, Unit Delay/1
  Sum/1 -> T/2/1

== system HybridControllerD3D3/dsp2acc/reference generator/integrator 2 ==
  inp : Inport
  Sum : Sum  Inputs=|++  SaturateOnIntegerOverflow=on  InputSameDT=on  OutDataTypeStr=Inherit: Same as first input
  Sum1 : Sum  Inputs=|++  SaturateOnIntegerOverflow=on  InputSameDT=on  OutDataTypeStr=Inherit: Same as first input
  T/2 : Gain  Gain=samplePeriod/2
  Unit Delay : UnitDelay  SampleTime=-1
  Unit Delay1 : UnitDelay  InitialCondition=initialCondition  SampleTime=-1
  out : Outport
  wires:
  T/2/1 -> Sum1/1
  Sum1/1 -> out/1, Unit Delay1/1
  Unit Delay1/1 -> Sum1/2
  Unit Delay/1 -> Sum/2
  inp/1 -> Sum/1, Unit Delay/1
  Sum/1 -> T/2/1

== system HybridControllerD3D3/xPC HC/Offset/If Action ==
  In1 : Inport
  Action Port : ActionPort  PropagateVarSize=During execution  ActionType=then
  Data Store Read : DataStoreRead  DataStoreName=x0  SampleTime=dt
  Data Store Write : DataStoreWrite  DataStoreName=x0
  Gain : Gain  Gain=1/nOffset  SaturateOnIntegerOverflow=on  OutDataTypeStr=Inherit: Same as input  ParamDataTypeStr=Inherit: Same as input
  Sum : Sum  Inputs=|++  SaturateOnIntegerOverflow=on  InputSameDT=on  OutDataTypeStr=Inherit: Same as first input
  wires:
  Data Store Read/1 -> Sum/2
  Sum/1 -> Data Store Write/1
  Gain/1 -> Sum/1
  In1/1 -> Gain/1

== system HybridControllerD3D3/xPC HC/Offset1/If Action ==
  In1 : Inport
  Action Port : ActionPort  PropagateVarSize=During execution  ActionType=then
  Data Store Read : DataStoreRead  DataStoreName=x0  SampleTime=dt
  Data Store Write : DataStoreWrite  DataStoreName=x0
  Gain : Gain  Gain=1/nOffset  SaturateOnIntegerOverflow=on  OutDataTypeStr=Inherit: Same as input  ParamDataTypeStr=Inherit: Same as input
  Sum : Sum  Inputs=|++  SaturateOnIntegerOverflow=on  InputSameDT=on  OutDataTypeStr=Inherit: Same as first input
  wires:
  Data Store Read/1 -> Sum/2
  Sum/1 -> Data Store Write/1
  Gain/1 -> Sum/1
  In1/1 -> Gain/1

== system HybridControllerD3D3/xPC HC/SubSystem0/If Action Subsystem0 ==
  Action Port : ActionPort  PropagateVarSize=During execution  ActionType=then
  Data Store Write0 : DataStoreWrite  DataStoreName=sFlag
  Data Store Write1 : DataStoreWrite  DataStoreName=tFlag
  atTargetFlag : Constant  Value=0  OutDataTypeStr=uint32  SampleTime=dtCon
  switchFlag : Constant  OutDataTypeStr=uint32  SampleTime=dtCon
  wires:
  atTargetFlag/1 -> Data Store Write1/1
  switchFlag/1 -> Data Store Write0/1

== system HybridControllerD3D3/xPC HC/SubSystem0/If Action Subsystem1 ==
  Action Port : ActionPort  PropagateVarSize=During execution  ActionType=then
  Data Store Write0 : DataStoreWrite  DataStoreName=sFlag
  switchFlag : Constant  Value=0  OutDataTypeStr=uint32  SampleTime=dtCon
  wires:
  switchFlag/1 -> Data Store Write0/1

== system HybridControllerD3D3/xPC HC/SubSystem1/SubSystem ==
  measDsp In : Inport
  measFrc In : Inport  Port=2
  Trigger : TriggerPort
  Data Store Write : DataStoreWrite  DataStoreName=tFlag
  atTargetFlag : Constant  OutDataTypeStr=uint32  SampleTime=-1
  measDsp Out : Outport  InitialOutput=[0]
  measFrc Out : Outport  Port=2  InitialOutput=[0]
  wires:
  atTargetFlag/1 -> Data Store Write/1
  measFrc In/1 -> measFrc Out/1
  measDsp In/1 -> measDsp Out/1

== system HybridControllerD3D3/xPC HC/SubSystem1/Subsystem ==
  i : Inport
  Add : Sum
  Constant : Constant  Value=iDelay
  Constant1 : Constant  Value=N
  If : If  IfExpression=u1 == 0
  If Action Subsystem1 : Subsystem  TreatAsAtomicUnit=on
  If Action Subsystem2 : Subsystem  TreatAsAtomicUnit=on
  trig : Outport
  wires:
  Constant/1 -> If/1, If Action Subsystem2/2(In2)
  If/1 -> If Action Subsystem1/Action
  If/2 -> If Action Subsystem2/Action
  If Action Subsystem1/1(Out1) -> Add/1
  If Action Subsystem2/1(Out1) -> Add/2
  Add/1 -> trig/1
  i/1 -> If Action Subsystem1/2(In2), If Action Subsystem2/1(In1)
  Constant1/1 -> If Action Subsystem1/1(In1)

== system HybridControllerD3D3/xPC HC/SubSystem1/Subsystem/If Action Subsystem1 ==
  In1 : Inport
  In2 : Inport  Port=2
  Action Port : ActionPort  PropagateVarSize=During execution  ActionType=then
  Relational Operator : RelationalOperator  Operator===  OutDataTypeStr=boolean
  Out1 : Outport
  wires:
  Relational Operator/1 -> Out1/1
  In1/1 -> Relational Operator/1
  In2/1 -> Relational Operator/2

== system HybridControllerD3D3/xPC HC/SubSystem1/Subsystem/If Action Subsystem2 ==
  In1 : Inport
  In2 : Inport  Port=2
  Action Port : ActionPort  PropagateVarSize=During execution  ActionType=else
  Relational Operator : RelationalOperator  Operator===  OutDataTypeStr=boolean
  Out1 : Outport
  wires:
  Relational Operator/1 -> Out1/1
  In1/1 -> Relational Operator/1
  In2/1 -> Relational Operator/2

== stateflow chart xPC HC/Predictor-Corrector ==
  state HybridController [parallel]
    settings: executionOrder=1
    state Predict
      en: state = 1;
      en: setCurDsp(com,i/N);
      en: diSD = 1;
      en: i = 1; iSD = 0;
      en: predictD3(com,i/N);
      du: i++;
      du: predictD3(com,i/N);
    state Initialize
      en: i = 1; iSD = 0;
      en: diSD = 1;
      en: initData(nAct,dtCon);
      en: zeroDsp(com);
    state AutoSlowDown
      en: state = 2;
      en: diSD = 4-i/(0.2*N);
      en: i += diSD; iSD = i;
      en: predictD3(com,i/N);
      du: diSD = 4-i/(0.2*N);
      du: i += diSD; iSD = i;
      du: predictD3(com,i/N);
    state Correct
      en: state = 0;
      en: setCurDsp(com,i/N);
      en: dspLocal = dsp; setNewDsp(dspLocal);
      en: di = min(max(diSD+1/(0.2*N)*(i-iSD),0.001),1.0);
      en: i = min(i+di,N);
      en: correctD3(com,i/N);
      du: di = min(max(diSD+1/(0.2*N)*(i-iSD),0.001),1.0);
      du: i = min(i+di,N);
      du: correctD3(com,i/N);
    Correct -> Predict : [i>=N]
    (default) -> Initialize
    Initialize -> Correct : [flag==1]
    AutoSlowDown -> Correct : [flag==1]
    Predict -> Correct [order 2] : [flag==1]
    Predict -> AutoSlowDown [order 1] : [i>=0.6*N && flag~=1]
  data: dsp input double size=nAct+1; flag input double size=1; com output double size=nAct+1; state output double size=1; i output double size=1; N local double size=1; nAct parameter double size=1 =1; di local double size=1; diSD local double size=1; iSD local double size=1; dspLocal local double size=nAct+1
